simulink model "practica_1_Simulink_II"  (R2018a)
settings: Solver=VariableStepAuto  StartTime=0.0  StopTime=100.0  RelTol=1e-3
values from neighbouring files (symbols this model uses):
  A_1 = 1    [Practica 1.3.m]    (also in practica1Parte2.m)
  a_1 = 0.1    [Practica 1.3.m]    (also in practica1Parte2.m)
  A_2 = 1    [Practica 1.3.m]    (also in practica1Parte2.m)
  a_2 = 0.1    [Practica 1.3.m]    (also in practica1Parte2.m)
  g = 9.81    [Practica 1.3.m]    (also in pactica1.m = 9.8; practica1Parte2.m)
  gamma = 0.6    [Practica 1.3.m]    (also in practica1Parte2.m)
settings Model: Creator=rafaelbeltranhernandez  LastModifiedBy=rafaelbeltranhernandez

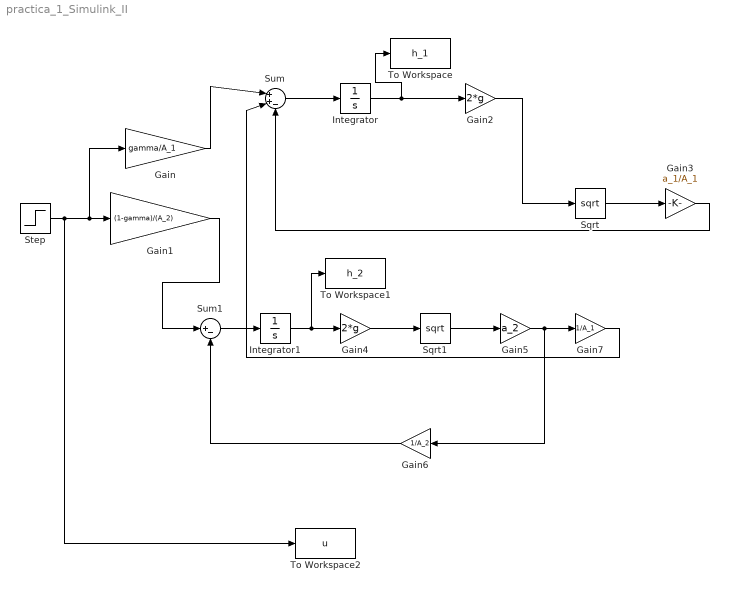
== system practica_1_Simulink_II ==
  Gain : Gain  Gain=gamma/A_1
  Gain1 : Gain  Gain=(1-gamma)/(A_2)
  Gain2 : Gain  Gain=2*g
  Gain3 : Gain  Gain=a_1/A_1
  Gain4 : Gain  Gain=2*g
  Gain5 : Gain  Gain=a_2
  Gain6 : Gain  Gain=1/A_2
  Gain7 : Gain  Gain=1/A_1
  Integrator : Integrator
  Integrator1 : Integrator
  Sqrt : Sqrt  SaturateOnIntegerOverflow=on
  Sqrt1 : Sqrt  SaturateOnIntegerOverflow=on
  Step : Step  After=0.44444  SampleTime=0
  Sum : Sum  Inputs=|++-
  Sum1 : Sum  Inputs=|+-
  To Workspace : ToWorkspace  VariableName=h_1  SaveFormat=Timeseries  SampleTime=-1
  To Workspace1 : ToWorkspace  VariableName=h_2  SaveFormat=Timeseries  SampleTime=-1
  To Workspace2 : ToWorkspace  VariableName=u  SaveFormat=Timeseries  SampleTime=-1
  wires:
  Step/1 -> To Workspace2/1, Gain/1, Gain1/1
  Gain/1 -> Sum/1
  Sum/1 -> Integrator/1
  Integrator/1 -> To Workspace/1, Gain2/1
  Gain2/1 -> Sqrt/1
  Sqrt/1 -> Gain3/1
  Gain3/1 -> Sum/3
  Gain1/1 -> Sum1/1
  Sum1/1 -> Integrator1/1
  Integrator1/1 -> To Workspace1/1, Gain4/1
  Gain4/1 -> Sqrt1/1
  Sqrt1/1 -> Gain5/1
  Gain5/1 -> Gain7/1, Gain6/1
  Gain6/1 -> Sum1/2
  Gain7/1 -> Sum/2
